simulink model "RudderActuatorChannel_check2"  (R2015a)
settings: Solver=ode4  StartTime=0.0  StopTime=2.999  FixedStep=1e-5  MaxStep=1e-3  MinStep=1e-4
undefined symbols (not defined in the file or in its folder): Acv, Aleak1, Aleak2, Aleak3, Aleak4, Aleak5, Aleakext, Aleakint, Ap, Ap_seal, Ar_seal, As_ehsv, Bkp_seal, Bp1, C, Cd, DeltaQ_ehsv, EHSV, EHSV_Step, EHSVFreqTest, EHSVTest, ent_air, frictionstribeck_velocity, i_ehsv, Input, K2_ehsv, K3_ehsv, K_Supply1, Ka1, Ki_ehsv, Kr_ehsv, ksi_ehsv, Kst, Kst_Enable, Kw_ehsv, L0, Load_cmd, Lp_seal, Lr_seal, Max_Cmd, Max_Load_TED, Max_Load_TEU, Mp1, P10, Pcvac, Pcvi, Pcvr, Ps0, Pt0, Ql_ehsv, R, Return_Pressure, Rho, seal_compression, seal_hardness, SealConstValue, SealType, sigbuilder_block, StiffnessTest_Enable, StiffTest ... (+15)
undefined symbols (not defined in the file): dpLVDT, ramLVDT, xvLVDT
libraries: simulink x1
(part 2 of 2)

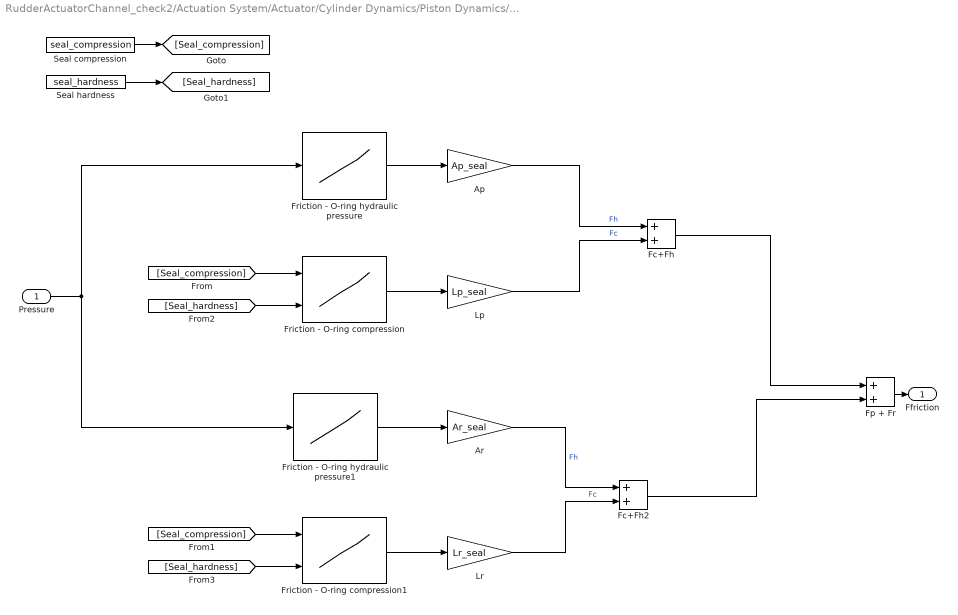
== system RudderActuatorChannel_check2/Actuation System/Actuator/Cylinder Dynamics/Piston Dynamics/Seal Friction Force/Force friction Piston+rod retraction ==
  Pressure : Inport
  Ap : Gain  Gain=Ap_seal
  Ar : Gain  Gain=Ar_seal
  Fc+Fh : Sum
  Fc+Fh2 : Sum
  Fp + Fr : Sum
  Friction - O-ring compression : Lookup_n-D  BreakpointsForDimension1=[0,5,10,15,20,25]  BreakpointsForDimension2=[70,80,90]  IndexSearchMethod=Linear search  Table=reshape([0,0.3,0.65,0.97313,1.37,1.7,0,0.6,1.22,1.82,2.45,3.05,0,0.8,1.6,2.37,3.2,3.98],6,3)  RndMeth=Simplest  InputSameDT=on
  Friction - O-ring compression1 : Lookup_n-D  BreakpointsForDimension1=[0,5,10,15,20,25]  BreakpointsForDimension2=[70,80,90]  IndexSearchMethod=Linear search  Table=reshape([0,0.3,0.65,0.97313,1.37,1.7,0,0.6,1.22,1.82,2.45,3.05,0,0.8,1.6,2.37,3.2,3.98],6,3)  RndMeth=Simplest  InputSameDT=on
  Friction - O-ring hydraulic pressure : Lookup_n-D  NumberOfTableDimensions=1  BreakpointsForDimension1=|  BreakpointsForDimension2=[70,80,90]  IndexSearchMethod=Linear search  Table=|  RndMeth=Simplest  InputSameDT=on
      BreakpointsForDimension1=|
      | [0
      | 500
      | 1000
      | 1500
      | 2000
      | 2500
      | 3000]
      Table=|
      | [0
      | 24.5
      | 37.5
      | 48
      | 58
      | 67
      | 72.1]
  Friction - O-ring hydraulic pressure1 : Lookup_n-D  NumberOfTableDimensions=1  BreakpointsForDimension1=|  BreakpointsForDimension2=[70,80,90]  IndexSearchMethod=Linear search  Table=|  RndMeth=Simplest  InputSameDT=on
      BreakpointsForDimension1=|
      | [0
      | 500
      | 1000
      | 1500
      | 2000
      | 2500
      | 3000]
      Table=|
      | [0
      | 24.5
      | 37.5
      | 48
      | 58
      | 67
      | 72.1]
  Lp : Gain  Gain=Lp_seal
  Lr : Gain  Gain=Lr_seal
  Seal compression : Constant  Value=seal_compression
  Seal hardness : Constant  Value=seal_hardness
  Ffriction : Outport
  wires:
  Friction - O-ring compression/1 -> Lp/1
  Lp/1 -> Fc+Fh/2  "Fc"
  Friction - O-ring hydraulic pressure/1 -> Ap/1
  Ap/1 -> Fc+Fh/1  "Fh"
  Fp + Fr/1 -> Ffriction/1
  Friction - O-ring compression1/1 -> Lr/1
  Lr/1 -> Fc+Fh2/2  "Fc"
  Pressure/1 -> Friction - O-ring hydraulic pressure/1, Friction - O-ring hydraulic pressure1/1
  Friction - O-ring hydraulic pressure1/1 -> Ar/1
  Ar/1 -> Fc+Fh2/1  "Fh"
  Fc+Fh2/1 -> Fp + Fr/2
  Fc+Fh/1 -> Fp + Fr/1
  Seal compression/1 -> [Seal_compression]
  [Seal_compression] -> Friction - O-ring compression/1
  [Seal_compression] -> Friction - O-ring compression1/1
  Seal hardness/1 -> [Seal_hardness]
  [Seal_hardness] -> Friction - O-ring compression/2
  [Seal_hardness] -> Friction - O-ring compression1/2

== system RudderActuatorChannel_check2/Actuation System/Actuator/Cylinder Dynamics/Piston Dynamics/Seal Friction Force/Stribeck effect ==
  Xp : Inport
  Abs : Abs
  Backlash : Backlash  BacklashWidth=.1
  Divide : Product  Inputs=*/
  Fcn : Fcn  Expr=exp(-u/frictionstribeck_velocity)
  Manual Switch : ManualSwitch  CurrentSetting=0
  Manual Switch1 : ManualSwitch  CurrentSetting=0
  Product : Product  RndMeth=Zero
  Stribeck factor : Outport
  wires:
  Xp/1 -> Manual Switch1/1, Backlash/1
  Abs/1 -> Divide/1, Fcn/1
  Fcn/1 -> Manual Switch/2, Product/2
  Divide/1 -> Product/1
  Product/1 -> Manual Switch/1
  Manual Switch/1 -> Stribeck factor/1
  Manual Switch1/1 -> Divide/2, Abs/1
  Backlash/1 -> Manual Switch1/2

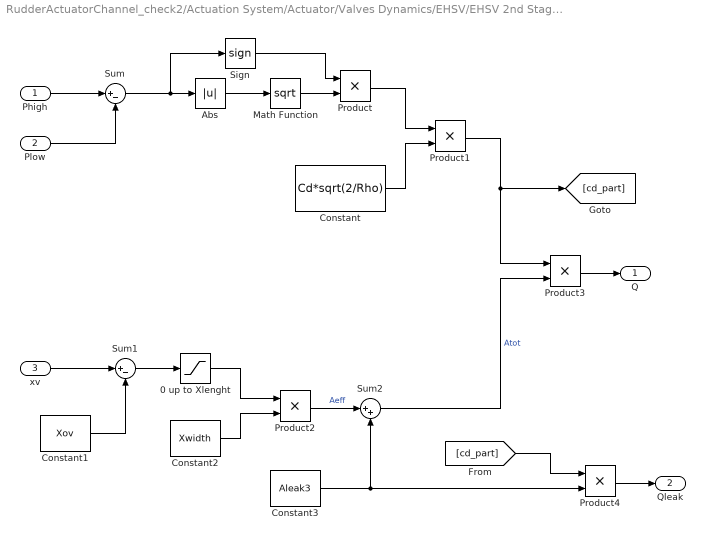
== system RudderActuatorChannel_check2/Actuation System/Actuator/Valves Dynamics/EHSV/EHSV 2nd Stage/C1 to R ==
  Phigh : Inport
  Plow : Inport  Port=2
  xv : Inport  Port=3
  0 up to Xlenght : Saturate  UpperLimit=Xlength  LowerLimit=0
  Abs : Abs
  Constant : Constant  Value=Cd*sqrt(2/Rho)
  Constant1 : Constant  Value=Xov
  Constant2 : Constant  Value=Xwidth
  Constant3 : Constant  Value=Aleak3
  Math Function : Math  Operator=sqrt  SaturateOnIntegerOverflow=on
  Product{,1..4} (5 alike) : Product  RndMeth=Zero
  Sign : Signum
  Sum : Sum  Inputs=|+-
  Sum1 : Sum  Inputs=|+-
  Sum2 : Sum  Inputs=|++
  Q : Outport
  Qleak : Outport  Port=2
  wires:
  Phigh/1 -> Sum/1
  Plow/1 -> Sum/2
  Sum/1 -> Abs/1, Sign/1
  Abs/1 -> Math Function/1
  Sign/1 -> Product/1
  Math Function/1 -> Product/2
  Constant/1 -> Product1/2
  Product/1 -> Product1/1
  xv/1 -> Sum1/1
  Constant1/1 -> Sum1/2
  Sum1/1 -> 0 up to Xlenght/1
  0 up to Xlenght/1 -> Product2/1
  Constant2/1 -> Product2/2
  Product2/1 -> Sum2/1  "Aeff"
  Constant3/1 -> Product4/2, Sum2/2
  Product1/1 -> [cd_part], Product3/1
  Sum2/1 -> Product3/2  "Atot"
  Product3/1 -> Q/1
  Product4/1 -> Qleak/1
  [cd_part] -> Product4/1

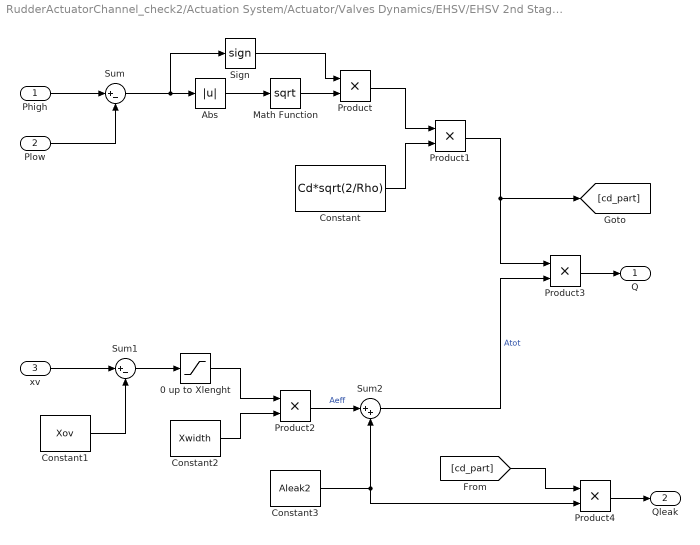
== system RudderActuatorChannel_check2/Actuation System/Actuator/Valves Dynamics/EHSV/EHSV 2nd Stage/C2 to R ==
  Phigh : Inport
  Plow : Inport  Port=2
  xv : Inport  Port=3
  0 up to Xlenght : Saturate  UpperLimit=Xlength  LowerLimit=0
  Abs : Abs
  Constant : Constant  Value=Cd*sqrt(2/Rho)
  Constant1 : Constant  Value=Xov
  Constant2 : Constant  Value=Xwidth
  Constant3 : Constant  Value=Aleak2
  Math Function : Math  Operator=sqrt  SaturateOnIntegerOverflow=on
  Product{,1..4} (5 alike) : Product  RndMeth=Zero
  Sign : Signum
  Sum : Sum  Inputs=|+-
  Sum1 : Sum  Inputs=|+-
  Sum2 : Sum  Inputs=|++
  Q : Outport
  Qleak : Outport  Port=2
  wires:
  Product3/1 -> Q/1
  Sum2/1 -> Product3/2  "Atot"
  Product1/1 -> [cd_part], Product3/1
  Product2/1 -> Sum2/1  "Aeff"
  Constant2/1 -> Product2/2
  0 up to Xlenght/1 -> Product2/1
  Sum1/1 -> 0 up to Xlenght/1
  Constant1/1 -> Sum1/2
  xv/1 -> Sum1/1
  Product/1 -> Product1/1
  Constant/1 -> Product1/2
  Math Function/1 -> Product/2
  Sign/1 -> Product/1
  Abs/1 -> Math Function/1
  Sum/1 -> Sign/1, Abs/1
  Plow/1 -> Sum/2
  Phigh/1 -> Sum/1
  Constant3/1 -> Product4/2, Sum2/2
  Product4/1 -> Qleak/1
  [cd_part] -> Product4/1

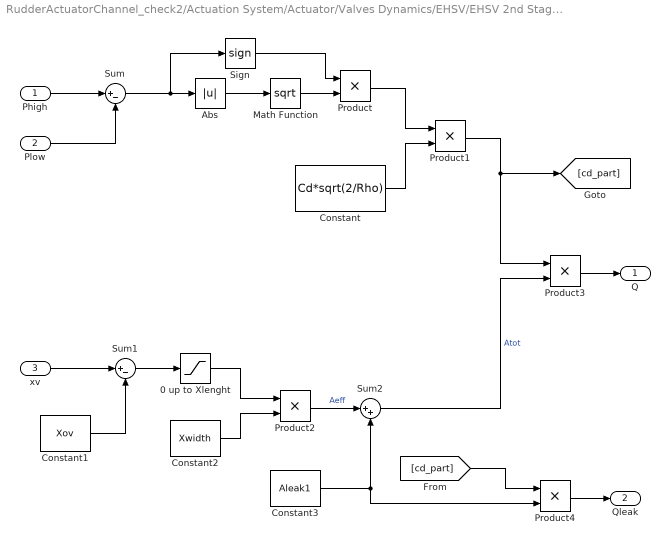
== system RudderActuatorChannel_check2/Actuation System/Actuator/Valves Dynamics/EHSV/EHSV 2nd Stage/P to C1 ==
  Phigh : Inport
  Plow : Inport  Port=2
  xv : Inport  Port=3
  0 up to Xlenght : Saturate  UpperLimit=Xlength  LowerLimit=0
  Abs : Abs
  Constant : Constant  Value=Cd*sqrt(2/Rho)
  Constant1 : Constant  Value=Xov
  Constant2 : Constant  Value=Xwidth
  Constant3 : Constant  Value=Aleak1
  Math Function : Math  Operator=sqrt  SaturateOnIntegerOverflow=on
  Product{,1..4} (5 alike) : Product  RndMeth=Zero
  Sign : Signum
  Sum : Sum  Inputs=|+-
  Sum1 : Sum  Inputs=|+-
  Sum2 : Sum  Inputs=|++
  Q : Outport
  Qleak : Outport  Port=2
  wires:
  Phigh/1 -> Sum/1
  Plow/1 -> Sum/2
  Sum/1 -> Abs/1, Sign/1
  Abs/1 -> Math Function/1
  Sign/1 -> Product/1
  Math Function/1 -> Product/2
  Constant/1 -> Product1/2
  Product/1 -> Product1/1
  xv/1 -> Sum1/1
  Constant1/1 -> Sum1/2
  Sum1/1 -> 0 up to Xlenght/1
  0 up to Xlenght/1 -> Product2/1
  Constant2/1 -> Product2/2
  Product2/1 -> Sum2/1  "Aeff"
  Constant3/1 -> Sum2/2, Product4/2
  Product1/1 -> [cd_part], Product3/1
  Sum2/1 -> Product3/2  "Atot"
  Product3/1 -> Q/1
  Product4/1 -> Qleak/1
  [cd_part] -> Product4/1

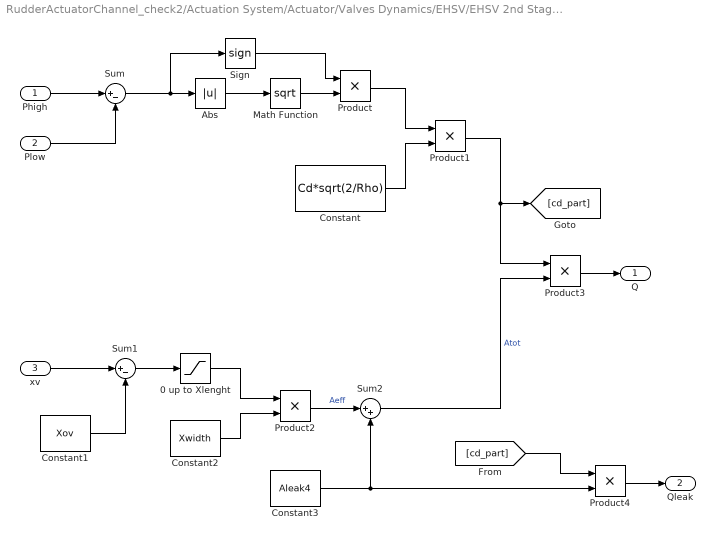
== system RudderActuatorChannel_check2/Actuation System/Actuator/Valves Dynamics/EHSV/EHSV 2nd Stage/P to C2 ==
  Phigh : Inport
  Plow : Inport  Port=2
  xv : Inport  Port=3
  0 up to Xlenght : Saturate  UpperLimit=Xlength  LowerLimit=0
  Abs : Abs
  Constant : Constant  Value=Cd*sqrt(2/Rho)
  Constant1 : Constant  Value=Xov
  Constant2 : Constant  Value=Xwidth
  Constant3 : Constant  Value=Aleak4
  Math Function : Math  Operator=sqrt  SaturateOnIntegerOverflow=on
  Product{,1..4} (5 alike) : Product  RndMeth=Zero
  Sign : Signum
  Sum : Sum  Inputs=|+-
  Sum1 : Sum  Inputs=|+-
  Sum2 : Sum  Inputs=|++
  Q : Outport
  Qleak : Outport  Port=2
  wires:
  Product3/1 -> Q/1
  Sum2/1 -> Product3/2  "Atot"
  Product1/1 -> [cd_part], Product3/1
  Product2/1 -> Sum2/1  "Aeff"
  Constant2/1 -> Product2/2
  0 up to Xlenght/1 -> Product2/1
  Sum1/1 -> 0 up to Xlenght/1
  Constant1/1 -> Sum1/2
  xv/1 -> Sum1/1
  Product/1 -> Product1/1
  Constant/1 -> Product1/2
  Math Function/1 -> Product/2
  Sign/1 -> Product/1
  Abs/1 -> Math Function/1
  Sum/1 -> Sign/1, Abs/1
  Plow/1 -> Sum/2
  Phigh/1 -> Sum/1
  Constant3/1 -> Sum2/2, Product4/2
  Product4/1 -> Qleak/1
  [cd_part] -> Product4/1

== system RudderActuatorChannel_check2/Actuation System/Actuator/Valves Dynamics/EHSV/EHSV 2nd Stage/P to R ==
  Phigh : Inport
  Plow : Inport  Port=2
  Abs : Abs
  Constant : Constant  Value=Cd*sqrt(2/Rho)
  Constant3 : Constant  Value=Aleak5
  Math Function : Math  Operator=sqrt  SaturateOnIntegerOverflow=on
  Product : Product  RndMeth=Zero
  Product1 : Product  RndMeth=Zero
  Product3 : Product  RndMeth=Zero
  Sign : Signum
  Sum : Sum  Inputs=|+-
  Q : Outport
  wires:
  Phigh/1 -> Sum/1
  Plow/1 -> Sum/2
  Sum/1 -> Abs/1, Sign/1
  Abs/1 -> Math Function/1
  Sign/1 -> Product/1
  Math Function/1 -> Product/2
  Constant/1 -> Product1/2
  Product/1 -> Product1/1
  Constant3/1 -> Product3/2  "Atot"
  Product1/1 -> Product3/1
  Product3/1 -> Q/1
